simulink model "SyntheticHDTVSimulation_CONOPS_Context"  (R2026a)
settings: Solver=VariableStepAuto
settings Model: Creator=pwilliam  LastModifiedBy=pwilliam

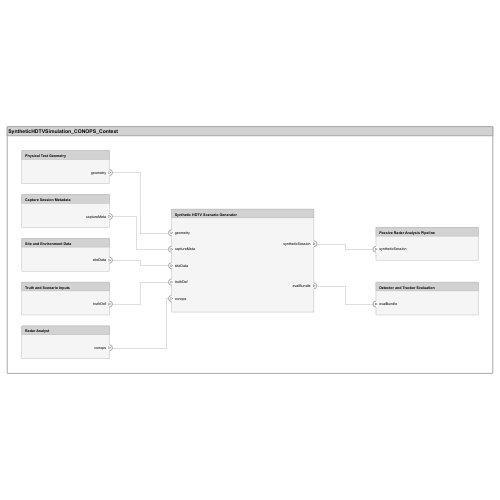
[thumbnail: Simulink's stored preview of the top-level diagram]
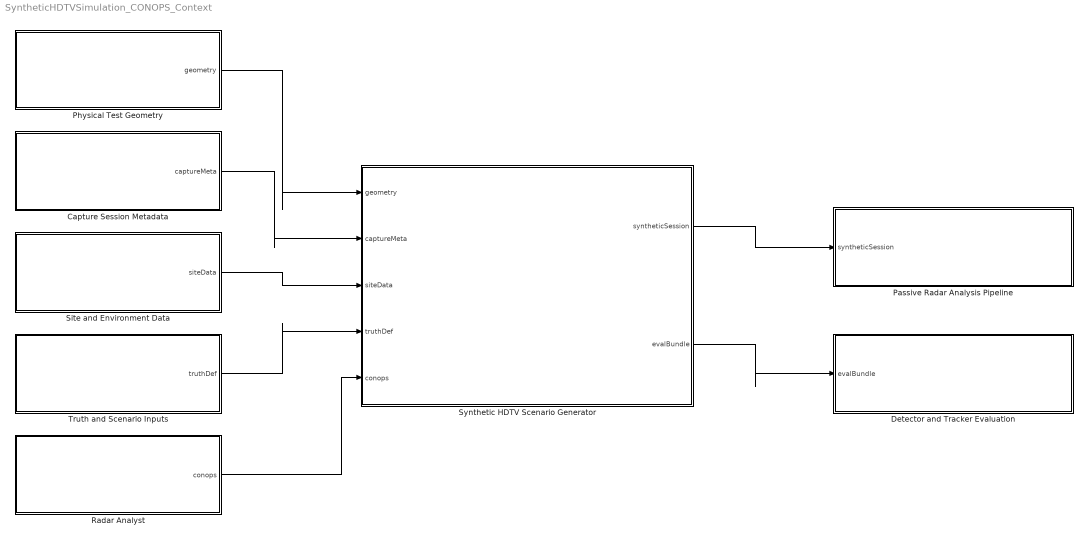
== system SyntheticHDTVSimulation_CONOPS_Context ==
  Capture Session Metadata : Subsystem
      settings: PortSchema="{\"entries\":[{\"content\":{\"headerSize\":26,\"margin\":15,\"minimumSpacing\":25,\"sides\":[{\"content\":{},\"type\":\"ConnectorPlacement.EquallySpacedRectSide\",\"uuid\":\"4300eb1c-d4d5-4905-8bef-bb51c5b7c80b\"},{\"content\":{\"connectorIds\":[\"Out1\"],\"side\":\"RIGHT\"},\"type\":\"ConnectorPlacement.EquallySpacedRectSide\",\"uuid\":\"a0fa5b78-ec46-44e0-b7e4-24e3bfc79eb1\"},{\"content\":{\"side\":\"TOP\"},\"type\":\"ConnectorPlacement.EquallySpacedRectSide\",\"uuid\":\"aa8d4c05-20a1-4f69-83d6-80dc021edc57\"}]},\"type\":\"ConnectorPlacement.EquallySpacedConnector\",\"uuid\":\"cd0e7431-6159-4193-8f53-5ead4c64d70c\"}],\"packageUris\":[\"http://schema.mathworks.com/mf0/Connector/R2020b\"],\"version\":\"1.0\"}"
  Detector and Tracker Evaluation : Subsystem
      settings: PortSchema="{\"entries\":[{\"content\":{\"headerSize\":26,\"margin\":15,\"minimumSpacing\":25,\"sides\":[{\"content\":{\"connectorIds\":[\"In1\"]},\"type\":\"ConnectorPlacement.EquallySpacedRectSide\",\"uuid\":\"4300eb1c-d4d5-4905-8bef-bb51c5b7c80b\"},{\"content\":{\"side\":\"RIGHT\"},\"type\":\"ConnectorPlacement.EquallySpacedRectSide\",\"uuid\":\"a0fa5b78-ec46-44e0-b7e4-24e3bfc79eb1\"},{\"content\":{\"side\":\"TOP\"},\"type\":\"ConnectorPlacement.EquallySpacedRectSide\",\"uuid\":\"aa8d4c05-20a1-4f69-83d6-80dc021edc57\"}]},\"type\":\"ConnectorPlacement.EquallySpacedConnector\",\"uuid\":\"cd0e7431-6159-4193-8f53-5ead4c64d70c\"}],\"packageUris\":[\"http://schema.mathworks.com/mf0/Connector/R2020b\"],\"version\":\"1.0\"}"
  Passive Radar Analysis Pipeline : Subsystem
      settings: PortSchema="{\"entries\":[{\"content\":{\"headerSize\":26,\"margin\":15,\"minimumSpacing\":25,\"sides\":[{\"content\":{\"connectorIds\":[\"In1\"]},\"type\":\"ConnectorPlacement.EquallySpacedRectSide\",\"uuid\":\"4300eb1c-d4d5-4905-8bef-bb51c5b7c80b\"},{\"content\":{\"side\":\"RIGHT\"},\"type\":\"ConnectorPlacement.EquallySpacedRectSide\",\"uuid\":\"a0fa5b78-ec46-44e0-b7e4-24e3bfc79eb1\"},{\"content\":{\"side\":\"TOP\"},\"type\":\"ConnectorPlacement.EquallySpacedRectSide\",\"uuid\":\"aa8d4c05-20a1-4f69-83d6-80dc021edc57\"}]},\"type\":\"ConnectorPlacement.EquallySpacedConnector\",\"uuid\":\"cd0e7431-6159-4193-8f53-5ead4c64d70c\"}],\"packageUris\":[\"http://schema.mathworks.com/mf0/Connector/R2020b\"],\"version\":\"1.0\"}"
  Physical Test Geometry : Subsystem
      settings: PortSchema="{\"entries\":[{\"content\":{\"headerSize\":26,\"margin\":15,\"minimumSpacing\":25,\"sides\":[{\"content\":{},\"type\":\"ConnectorPlacement.EquallySpacedRectSide\",\"uuid\":\"4300eb1c-d4d5-4905-8bef-bb51c5b7c80b\"},{\"content\":{\"connectorIds\":[\"Out1\"],\"side\":\"RIGHT\"},\"type\":\"ConnectorPlacement.EquallySpacedRectSide\",\"uuid\":\"a0fa5b78-ec46-44e0-b7e4-24e3bfc79eb1\"},{\"content\":{\"side\":\"TOP\"},\"type\":\"ConnectorPlacement.EquallySpacedRectSide\",\"uuid\":\"aa8d4c05-20a1-4f69-83d6-80dc021edc57\"}]},\"type\":\"ConnectorPlacement.EquallySpacedConnector\",\"uuid\":\"cd0e7431-6159-4193-8f53-5ead4c64d70c\"}],\"packageUris\":[\"http://schema.mathworks.com/mf0/Connector/R2020b\"],\"version\":\"1.0\"}"
  Radar Analyst : Subsystem
      settings: PortSchema="{\"entries\":[{\"content\":{\"headerSize\":26,\"margin\":15,\"minimumSpacing\":25,\"sides\":[{\"content\":{},\"type\":\"ConnectorPlacement.EquallySpacedRectSide\",\"uuid\":\"4300eb1c-d4d5-4905-8bef-bb51c5b7c80b\"},{\"content\":{\"connectorIds\":[\"Out1\"],\"side\":\"RIGHT\"},\"type\":\"ConnectorPlacement.EquallySpacedRectSide\",\"uuid\":\"a0fa5b78-ec46-44e0-b7e4-24e3bfc79eb1\"},{\"content\":{\"side\":\"TOP\"},\"type\":\"ConnectorPlacement.EquallySpacedRectSide\",\"uuid\":\"aa8d4c05-20a1-4f69-83d6-80dc021edc57\"}]},\"type\":\"ConnectorPlacement.EquallySpacedConnector\",\"uuid\":\"cd0e7431-6159-4193-8f53-5ead4c64d70c\"}],\"packageUris\":[\"http://schema.mathworks.com/mf0/Connector/R2020b\"],\"version\":\"1.0\"}"
  Site and Environment Data : Subsystem
      settings: PortSchema="{\"entries\":[{\"content\":{\"headerSize\":26,\"margin\":15,\"minimumSpacing\":25,\"sides\":[{\"content\":{},\"type\":\"ConnectorPlacement.EquallySpacedRectSide\",\"uuid\":\"4300eb1c-d4d5-4905-8bef-bb51c5b7c80b\"},{\"content\":{\"connectorIds\":[\"Out1\"],\"side\":\"RIGHT\"},\"type\":\"ConnectorPlacement.EquallySpacedRectSide\",\"uuid\":\"a0fa5b78-ec46-44e0-b7e4-24e3bfc79eb1\"},{\"content\":{\"side\":\"TOP\"},\"type\":\"ConnectorPlacement.EquallySpacedRectSide\",\"uuid\":\"aa8d4c05-20a1-4f69-83d6-80dc021edc57\"}]},\"type\":\"ConnectorPlacement.EquallySpacedConnector\",\"uuid\":\"cd0e7431-6159-4193-8f53-5ead4c64d70c\"}],\"packageUris\":[\"http://schema.mathworks.com/mf0/Connector/R2020b\"],\"version\":\"1.0\"}"
  Synthetic HDTV Scenario Generator : Subsystem
      settings: PortSchema="{\"entries\":[{\"content\":{\"headerSize\":26,\"margin\":15,\"minimumSpacing\":25,\"sides\":[{\"content\":{\"connectorIds\":[\"In1\",\"In2\",\"In3\",\"In4\",\"In5\"]},\"type\":\"ConnectorPlacement.EquallySpacedRectSide\",\"uuid\":\"4300eb1c-d4d5-4905-8bef-bb51c5b7c80b\"},{\"content\":{\"connectorIds\":[\"Out1\",\"Out2\"],\"side\":\"RIGHT\"},\"type\":\"ConnectorPlacement.EquallySpacedRectSide\",\"uuid\":\"a0fa5b78-ec46-44e0-b7e4-24e3bfc79eb1\"},{\"content\":{\"side\":\"TOP\"},\"type\":\"ConnectorPlacement.EquallySpacedRectSide\",\"uuid\":\"aa8d4c05-20a1-4f69-83d6-80dc021edc57\"}]},\"type\":\"ConnectorPlacement.EquallySpacedConnector\",\"uuid\":\"cd0e7431-6159-4193-8f53-5ead4c64d70c\"}],\"packageUris\":[\"http://schema.mathworks.com/mf0/Connector/R2020b\"],\"version\":\"1.0\"}"
  Truth and Scenario Inputs : Subsystem
      settings: PortSchema="{\"entries\":[{\"content\":{\"headerSize\":26,\"margin\":15,\"minimumSpacing\":25,\"sides\":[{\"content\":{},\"type\":\"ConnectorPlacement.EquallySpacedRectSide\",\"uuid\":\"4300eb1c-d4d5-4905-8bef-bb51c5b7c80b\"},{\"content\":{\"connectorIds\":[\"Out1\"],\"side\":\"RIGHT\"},\"type\":\"ConnectorPlacement.EquallySpacedRectSide\",\"uuid\":\"a0fa5b78-ec46-44e0-b7e4-24e3bfc79eb1\"},{\"content\":{\"side\":\"TOP\"},\"type\":\"ConnectorPlacement.EquallySpacedRectSide\",\"uuid\":\"aa8d4c05-20a1-4f69-83d6-80dc021edc57\"}]},\"type\":\"ConnectorPlacement.EquallySpacedConnector\",\"uuid\":\"cd0e7431-6159-4193-8f53-5ead4c64d70c\"}],\"packageUris\":[\"http://schema.mathworks.com/mf0/Connector/R2020b\"],\"version\":\"1.0\"}"
  wires:
  Physical Test Geometry/1(geometry) -> Synthetic HDTV Scenario Generator/1(geometry)
  Capture Session Metadata/1(captureMeta) -> Synthetic HDTV Scenario Generator/2(captureMeta)
  Site and Environment Data/1(siteData) -> Synthetic HDTV Scenario Generator/3(siteData)
  Truth and Scenario Inputs/1(truthDef) -> Synthetic HDTV Scenario Generator/4(truthDef)
  Radar Analyst/1(conops) -> Synthetic HDTV Scenario Generator/5(conops)
  Synthetic HDTV Scenario Generator/1(syntheticSession) -> Passive Radar Analysis Pipeline/1(syntheticSession)
  Synthetic HDTV Scenario Generator/2(evalBundle) -> Detector and Tracker Evaluation/1(evalBundle)

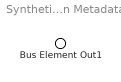
== system SyntheticHDTVSimulation_CONOPS_Context/Capture Session Metadata ==
  Bus Element Out1 : Outport  PortName=captureMeta

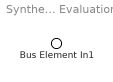
== system SyntheticHDTVSimulation_CONOPS_Context/Detector and Tracker Evaluation ==
  Bus Element In1 : Inport  PortName=evalBundle

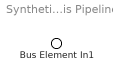
== system SyntheticHDTVSimulation_CONOPS_Context/Passive Radar Analysis Pipeline ==
  Bus Element In1 : Inport  PortName=syntheticSession

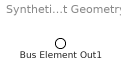
== system SyntheticHDTVSimulation_CONOPS_Context/Physical Test Geometry ==
  Bus Element Out1 : Outport  PortName=geometry

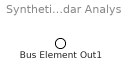
== system SyntheticHDTVSimulation_CONOPS_Context/Radar Analyst ==
  Bus Element Out1 : Outport  PortName=conops

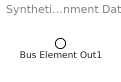
== system SyntheticHDTVSimulation_CONOPS_Context/Site and Environment Data ==
  Bus Element Out1 : Outport  PortName=siteData

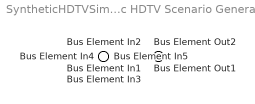
== system SyntheticHDTVSimulation_CONOPS_Context/Synthetic HDTV Scenario Generator ==
  Bus Element In1 : Inport  PortName=geometry
  Bus Element In2 : Inport  Port=2  PortName=captureMeta
  Bus Element In3 : Inport  Port=3  PortName=siteData
  Bus Element In4 : Inport  Port=4  PortName=truthDef
  Bus Element In5 : Inport  Port=5  PortName=conops
  Bus Element Out1 : Outport  PortName=syntheticSession
  Bus Element Out2 : Outport  Port=2  PortName=evalBundle

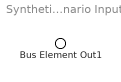
== system SyntheticHDTVSimulation_CONOPS_Context/Truth and Scenario Inputs ==
  Bus Element Out1 : Outport  PortName=truthDef
